simulink model "oscillatory"  (R2021b)
settings: Solver=VariableStepAuto  StartTime=0.0  StopTime=5  RelTol=1e-3
libraries: slctrlblks x1
settings Model: Creator=iliya122  LastModifiedBy=Ivan
settings SolverCC: AlgebraicLoopSolver=TrustRegion
settings DebuggingCC: SFMachineParentedDataDiag=warning

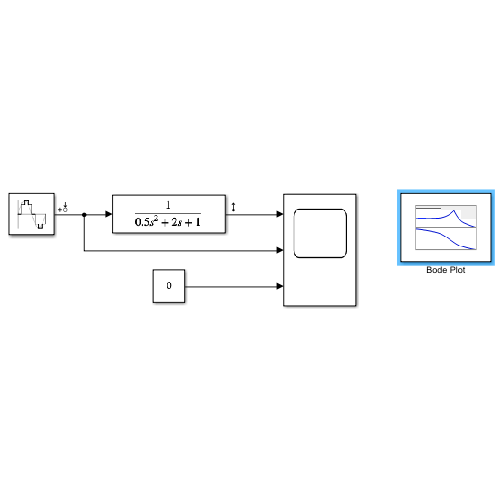
[thumbnail: Simulink's stored preview of the top-level diagram]
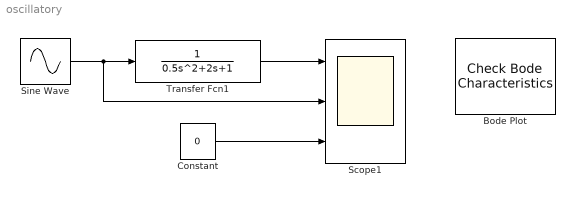
== system oscillatory ==
  Bode Plot : slctrlblks/Model Verification/Check Bode  Characteristics  InstantiateOnLoad=on  SaveOperatingPoints=off  LinearizationIOs={'/Sine Wave', 1, 'in', 'off', '';'/Transfer Fcn1', 1, 'out', 'off', ''}  LinearizeAt=SnapshotTimes  SnapshotTimes=[0]  TriggerType=rising  SampleTime=auto  RateConversionMethod=zoh  PreWarpFreq=10  UseExactDelayModel=off  UseFullBlockNameLabels=off  UseBusSignalLabels=off  enabled=on  stopWhenAssertionFail=off  export=off  ViewDlgPos=[404 121 1173 689]  OpenViewOnLoad=off  LaunchViewOnOpen=off  FrequencyUnits=rad/s  MagnitudeUnits=dB  PhaseUnits=deg  TimeUnits=seconds  EnableUpperBound=off  UpperBoundFrequencies=[]  UpperBoundMagnitudes=[]  EnableLowerBound=off  LowerBoundFrequencies=[]  LowerBoundMagnitudes=[]
  Constant : Constant  Value=0
  Scope1 : Scope  NumInputPorts=3
  Sine Wave : Sin  Frequency=10*(2*pi)  SampleTime=0.001
  Transfer Fcn1 : TransferFcn  Numerator=1  Denominator=[0.5 2 1]
  wires:
  Sine Wave/1 -> Scope1/2, Transfer Fcn1/1
  Constant/1 -> Scope1/3
  Transfer Fcn1/1 -> Scope1/1
